simulink model "TEST_LIDAR"  (R2022b)
settings: Solver=FixedStepAuto  StartTime=0.0  StopTime=inf  FixedStep=1e-3  RelTol=1e-3  EnableMultiTasking=on
model workspace (MAT data in the model file):
  SL_ROS_VariableLengthArrays_MaxSizes.CommonInfo.ArrayTruncateAction = 'EmitWarning'
  SL_ROS_VariableLengthArrays_MaxSizes.MsgTypeMap = containers.Map
  SL_ROS_VariableLengthArrays_MaxSizes.MsgTypeMap.serialization.keys = {'sensor_msgs/LaserScan', 'time_custom_msgs/Tiempos'}
  SL_ROS_VariableLengthArrays_MaxSizes.MsgTypeMap.serialization.values{1}(1).PropertyName = 'intensities'
  SL_ROS_VariableLengthArrays_MaxSizes.MsgTypeMap.serialization.values{1}(1).DataType = 'single'
  SL_ROS_VariableLengthArrays_MaxSizes.MsgTypeMap.serialization.values{1}(1).MaxLength = 128
  SL_ROS_VariableLengthArrays_MaxSizes.MsgTypeMap.serialization.values{1}(2).PropertyName = 'ranges'
  SL_ROS_VariableLengthArrays_MaxSizes.MsgTypeMap.serialization.values{1}(2).DataType = 'single'
  SL_ROS_VariableLengthArrays_MaxSizes.MsgTypeMap.serialization.values{1}(2).MaxLength = 1
  SL_ROS_VariableLengthArrays_MaxSizes.MsgTypeMap.serialization.values{2}.PropertyName = 'data'
  SL_ROS_VariableLengthArrays_MaxSizes.MsgTypeMap.serialization.values{2}.DataType = 'uint8'
  SL_ROS_VariableLengthArrays_MaxSizes.MsgTypeMap.serialization.values{2}.MaxLength = 1400
  SL_ROS_VariableLengthArrays_MaxSizes.MsgTypeMap.serialization.uniformity = 0
  SL_ROS_VariableLengthArrays_MaxSizes.MsgTypeMap.serialization.keyType = 'char'
  SL_ROS_VariableLengthArrays_MaxSizes.MsgTypeMap.serialization.valueType = 'any'
values from neighbouring files (symbols this model uses):
  data = theClient.GetLastFrameOfData()    [FuncMotive.m]
undefined symbols (not defined in the file or in its folder): angular, carstamp, CIRCUIT, CLTF_DAMP, CLTF_FREQ, CLTF_GAIN, CONTROL, CONTROL_INI, DiscIntNeverNeededParam, INPUT, linear, MCP3201, MD25, MODEL, MODEL_INI, mpcstate, MPU60X0, MPU9250, MSG, NAV_MPC_CONTROL, OUTPUT, RCRX, SAMPLING_TIME, SYSID_INPUT, VL6180X
libraries: raspberrypiCommlib x160, simulink x89, raspberrypiNetworklib x22, ros2lib x14, dspsigattribs x14, embedlinuxBasiclib x12, ctrlSharedLib x2, mpclib x1, vrlib x1, sldrtlib x1
(part 1 of 19)
settings Model: SimulationMode=external  PauseTimes=430  ExtModeTrigDuration=2  Creator=The MathWorks, Inc.  LastModifiedBy=diego
settings SolverCC: AlgebraicLoopSolver=TrustRegion  PositivePriorityOrder=on  AutoInsertRateTranBlk=on
settings DataIOCC: LimitDataPoints=on  SaveOutput=off  SignalLogging=off  DSMLogging=off  SaveTime=off  ReturnWorkspaceOutputs=off
settings OptimizationCC: BlockReduction=off  EnhancedBackFolding=on  PassReuseOutputArgsAs=Individual arguments  ZeroExternalMemoryAtStartup=off  ZeroInternalMemoryAtStartup=off  MaxStackSize=64  OptimizeBlockOrder=speed  DifferentSizesBufferReuse=on  OptimizationCustomize=off  EfficientTunableParamExpr=on
settings DebuggingCC: MultiTaskDSMMsg=none  ParameterPrecisionLossMsg=none  ParameterTunabilityLossMsg=error  UnconnectedInputMsg=warning  UnconnectedOutputMsg=warning  UnconnectedLineMsg=warning  AllowSymbolicDim=off  PregeneratedLibrarySubsystemCodeDiagnostic=none  SFUnexpectedBacktrackingDiag=warning  SFNoUnconditionalDefaultTransitionDiag=warning  SFExecutionAtInitializationDiag=none  SFMachineParentedDataDiag=warning  ArithmeticOperatorsInVariantConditions=warning
settings HardwareCC: ProdBitPerPointer=32  ProdBitPerSizeT=32  ProdBitPerPtrDiffT=32  ProdLargestAtomicInteger=Long  ProdLargestAtomicFloat=Double  ProdWordSize=32  ProdLongLongMode=on  ProdHWDeviceType=ARM Compatible->ARM Cortex
settings ModelReferenceCC: EnableRefExpFcnMdlSchedulingChecks=on  PropagateSignalLabelsOutOfModel=off
settings SFSimCC: SimUseLocalCustomCode=off  CustomCodeUndefinedFunction=UseInterfaceOnly
settings RTWCC: Description=Embedded Coder  SystemTargetFile=ert.tlc  HardwareBoard=Raspberry Pi  TemplateMakefile=ert_default_tmf  RTWUseLocalCustomCode=off  Toolchain=GNU GCC Embedded Linux  BuildConfiguration=Faster Runs  DLArmComputeVersion=19.05
settings CodeAppCC: ForceParamTrailComments=on  IgnoreCustomStorageClasses=off  MaxIdLength=95  OperatorAnnotations=on  SimulinkDataObjDesc=on  SFDataObjDesc=on  MangleLength=10  InsertBlockDesc=on
settings ERTTargetCC: SupportVariableSizeSignals=on  ExtMode=on  ExtModeTransport=2  ExtModeStaticAlloc=on  ExtModeMexFile=ext_xcp  ExtModeMexArgs='192.168.0.103' 0 17725  ExtModeIntrfLevel=Level2 - Open
settings ConfigComp: CovMetricSettings=dw  CovSaveCumulativeToWorkspaceVar=on  CovSaveSingleToWorkspaceVar=on  CovExternalEMLEnable=off

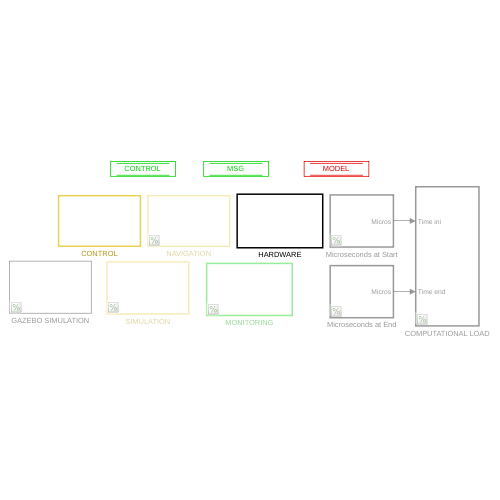
[thumbnail: Simulink's stored preview of the top-level diagram]
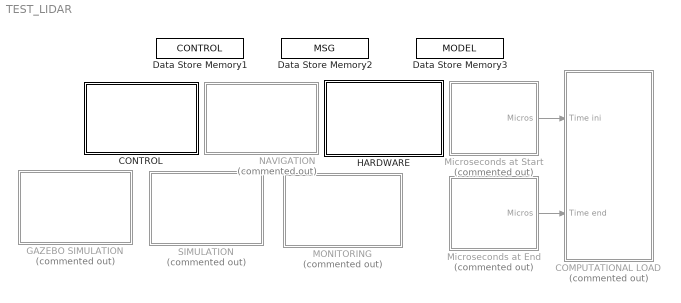
== system TEST_LIDAR ==
  COMPUTATIONAL LOAD : Subsystem  Priority=1100  Commented=on  TreatAsAtomicUnit=on  mask{Ts=SAMPLING_TIME}
      mask prompts: Ts "Sampling Time (s)"
      settings: MinAlgLoopOccurrences=on
  CONTROL : Subsystem  Priority=30  TreatAsAtomicUnit=on
      settings: MinAlgLoopOccurrences=on  RTWSystemCode=Nonreusable function  RTWFcnNameOpts=Use subsystem name  RTWFileNameOpts=Use subsystem name  FunctionWithSeparateData=on
  Data Store Memory1 : DataStoreMemory  Priority=2  DataStoreName=CONTROL  ReadBeforeWriteMsg=warning  WriteAfterWriteMsg=warning  WriteAfterReadMsg=warning  InitialValue=CONTROL_INI  ShowAdditionalParam=off  OutDataTypeStr=Bus: CONTROL_Bus
  Data Store Memory2 : DataStoreMemory  Priority=2  DataStoreName=MSG  ReadBeforeWriteMsg=warning  WriteAfterWriteMsg=warning  WriteAfterReadMsg=warning  InitialValue=MSG_INI  ShowAdditionalParam=off  OutDataTypeStr=Bus: MSG_Bus
  Data Store Memory3 : DataStoreMemory  Priority=2  DataStoreName=MODEL  ReadBeforeWriteMsg=warning  WriteAfterWriteMsg=warning  WriteAfterReadMsg=warning  InitialValue=MODEL_INI  ShowAdditionalParam=off  OutDataTypeStr=Bus: MODEL_Bus
  GAZEBO SIMULATION : Subsystem  Commented=on
  HARDWARE : Subsystem  Priority=10  TreatAsAtomicUnit=on
      settings: MinAlgLoopOccurrences=on
  MONITORING : Subsystem  Priority=100  Commented=on  TreatAsAtomicUnit=on
      settings: MinAlgLoopOccurrences=on
  Microseconds at End : Subsystem  Priority=1000  Commented=on  TreatAsAtomicUnit=on
      settings: MinAlgLoopOccurrences=on
  Microseconds at Start : Subsystem  Priority=0  Commented=on  TreatAsAtomicUnit=on
      settings: MinAlgLoopOccurrences=on
  NAVIGATION : Subsystem  Priority=30  Commented=on  TreatAsAtomicUnit=on
      settings: MinAlgLoopOccurrences=on  RTWSystemCode=Nonreusable function  RTWFcnNameOpts=Use subsystem name  RTWFileNameOpts=Use subsystem name  FunctionWithSeparateData=on
  SIMULATION : Subsystem  Priority=10  Commented=on  TreatAsAtomicUnit=on
      settings: MinAlgLoopOccurrences=on
  wires:
  Microseconds at End/1(Micros) -> COMPUTATIONAL LOAD/2(Time end)
  Microseconds at Start/1(Micros) -> COMPUTATIONAL LOAD/1(Time ini)

== system TEST_LIDAR/COMPUTATIONAL LOAD ==
  Time ini : Inport
  Time end : Inport  Port=2
  Accumulator 1 : Subsystem
  Accumulator 2 : Subsystem
  Accumulator 3 : Subsystem
  Accumulator 4 : Subsystem
  CPU Utilization (%) : Display
  CPU time (s) : Display
  Compare To Constant : simulink/Logic and Bit Operations/Compare To Constant  relop=>=  const=100  OutDataTypeStr=uint8
  Compare To Constant1 : simulink/Logic and Bit Operations/Compare To Constant  relop=>=  const=0  OutDataTypeStr=uint8
  Compare To Constant2 : simulink/Logic and Bit Operations/Compare To Constant  relop=<  const=0  OutDataTypeStr=uint8
  Cycles : Display
  Cycles Over 100% : Display
  Data Store Write : DataStoreWrite  DataStoreName=CONTROL  DataStoreElements=CONTROL.STATE.CPU_LOAD  IndexOptions=Index vector (dialog)  Indices=1  OutputSizes=1
  Data Type Conversion : DataTypeConversion  OutDataTypeStr=single  SaturateOnIntegerOverflow=off  RndMeth=Floor
  Data Type Conversion1 : DataTypeConversion  OutDataTypeStr=single  SaturateOnIntegerOverflow=off  RndMeth=Floor
  Data Type Conversion3 : DataTypeConversion  OutDataTypeStr=uint8  SaturateOnIntegerOverflow=off  RndMeth=Floor
  Gain : Gain  Gain=1e-4/Ts
  Gain1 : Gain  Gain=1e6
  Gain2 : Gain  Gain=1e3
  Mux2 : Mux  Inputs=2
  "Probably, priority error or time overflow" : Display
  Sum : Sum  Inputs=-|+  OutDataTypeStr=double
  usecs per Ts : Constant  Value=Ts*1e6  SampleTime=Ts
  wires:
  usecs per Ts/1 -> Accumulator 1/1(In)
  Sum/1 -> Gain/1
  Time ini/1 -> Gain2/1, Sum/1
  Accumulator 1/1(Sum) -> Gain1/1
  Accumulator 3/1(Sum) -> Cycles/1
  Compare To Constant1/1 -> Accumulator 3/1(In)
  Accumulator 2/1(Sum) -> Cycles Over 100%/1
  Compare To Constant/1 -> Accumulator 2/1(In)
  Time end/1 -> Sum/2
  Gain/1 -> CPU Utilization (%)/1, Data Type Conversion3/1, Compare To Constant/1, Compare To Constant2/1, Compare To Constant1/1
  Compare To Constant2/1 -> Accumulator 4/1(In)
  Accumulator 4/1(Sum) -> "Probably, priority error or time overflow"/1
  Gain1/1 -> Data Type Conversion/1
  Gain2/1 -> Data Type Conversion1/1
  Data Type Conversion/1 -> Mux2/1
  Data Type Conversion1/1 -> Mux2/2
  Mux2/1 -> CPU time (s)/1
  Data Type Conversion3/1 -> Data Store Write/1

== system TEST_LIDAR/CONTROL ==
  ACCELERATION RATE : Subsystem  Priority=50  Commented=on  TreatAsAtomicUnit=on
      settings: MinAlgLoopOccurrences=on
  ADAPTIVE CONTROL STR : Subsystem  Priority=200  Commented=on
      settings: MinAlgLoopOccurrences=on
  "CONTROL UPDATE " : MATLAB Function  Priority=30  Commented=on  TreatAsAtomicUnit=on
      settings: MinAlgLoopOccurrences=on
  Compare To Constant4 : simulink/Logic and Bit Operations/Compare To Constant  Commented=on  relop=>  const=0  OutDataTypeStr=boolean
  Compare To Constant9 : simulink/Logic and Bit Operations/Compare To Constant  Commented=on  relop===  const=5  OutDataTypeStr=boolean
  Data Store Read1 : DataStoreRead  Commented=on  DataStoreName=CONTROL  SampleTime=SAMPLING_TIME  IndexOptions=Index vector (dialog)  Indices=1  OutputSizes=1
  Data Store Read10 : DataStoreRead  Commented=on  DataStoreName=CONTROL  SampleTime=SAMPLING_TIME  DataStoreElements=CONTROL.OUTPUT.MOTOR_VOLT(:,:)  IndexOptions=Index vector (dialog)  Indices=1  OutputSizes=1
  Data Store Read11 : DataStoreRead  Commented=on  DataStoreName=CONTROL  SampleTime=SAMPLING_TIME  DataStoreElements=CONTROL.INPUT.BATTERY_VOLT  IndexOptions=Index vector (dialog)  Indices=1  OutputSizes=1
  Data Store Read2 : DataStoreRead  Commented=on  DataStoreName=CONTROL  SampleTime=SAMPLING_TIME  IndexOptions=Index vector (dialog)  Indices=1  OutputSizes=1
  Data Store Read5 : DataStoreRead  DataStoreName=MSG  SampleTime=SAMPLING_TIME  IndexOptions=Index vector (dialog)  Indices=1  OutputSizes=1
  Data Store Read6 : DataStoreRead  Commented=on  DataStoreName=CONTROL  SampleTime=SAMPLING_TIME  DataStoreElements=CONTROL.STATE.CURRENT_STATUS_SYS  IndexOptions=Index vector (dialog)  Indices=1  OutputSizes=1
  Data Store Read7 : DataStoreRead  DataStoreName=CONTROL  SampleTime=SAMPLING_TIME  IndexOptions=Index vector (dialog)  Indices=1  OutputSizes=1
  Data Store Read8 : DataStoreRead  Commented=on  DataStoreName=CONTROL  SampleTime=SAMPLING_TIME  DataStoreElements=CONTROL.STATE.STR_MODE  IndexOptions=Index vector (dialog)  Indices=1  OutputSizes=1
  Data Store Read9 : DataStoreRead  Commented=on  DataStoreName=CONTROL  SampleTime=SAMPLING_TIME  DataStoreElements=CONTROL.STATE.CONTROL_STATUS  IndexOptions=Index vector (dialog)  Indices=1  OutputSizes=1
  Data Store Write : DataStoreWrite  Commented=on  DataStoreName=CONTROL  DataStoreElements=CONTROL.OUTPUT.REAL_MOTOR_VOLT(:,:)  IndexOptions=Index vector (dialog)  Indices=1  OutputSizes=1
  Data Store Write1 : DataStoreWrite  Commented=on  DataStoreName=CONTROL  IndexOptions=Index vector (dialog)  Indices=1  OutputSizes=1
  Data Store Write2 : DataStoreWrite  Commented=on  DataStoreName=CONTROL  IndexOptions=Index vector (dialog)  Indices=1  OutputSizes=1
  Data Store Write3 : DataStoreWrite  DataStoreName=CONTROL  IndexOptions=Index vector (dialog)  Indices=1  OutputSizes=1
  Data Store Write5 : DataStoreWrite  DataStoreName=MSG  IndexOptions=Index vector (dialog)  Indices=1  OutputSizes=1
  Data Store Write6 : DataStoreWrite  Commented=on  DataStoreName=CONTROL  DataStoreElements=CONTROL.OUTPUT.REAL_MOTOR_VOLT_CD(:,:)  IndexOptions=Index vector (dialog)  Indices=1  OutputSizes=1
  LOCAL TARGETS : Subsystem  Priority=5  Commented=on  TreatAsAtomicUnit=on
      settings: MinAlgLoopOccurrences=on
  Logical Operator1 : Logic  Commented=on  AllPortsSameDT=off  OutDataTypeStr=boolean
  MOTOR DELAY : Subsystem  Priority=40  Commented=on  TreatAsAtomicUnit=on
      settings: MinAlgLoopOccurrences=on
  STATE ESTIMATOR : MATLAB Function  Priority=20  Commented=on  TreatAsAtomicUnit=on
      settings: MinAlgLoopOccurrences=on
  STATE MACHINE UPDATE : MATLAB Function  Priority=1000  TreatAsAtomicUnit=on
      settings: MinAlgLoopOccurrences=on
  SYSTEM IDENTIFICATION : Subsystem  Priority=150  Commented=on  TreatAsAtomicUnit=on
      mask init:
      | %%%%%%%%%%%%%%%%%%%%%%%%%%%%%%%%%%%%%%%%%%%%%%%%%%%%%%
      | %%  STATE VARIABLE FILTER FOR SYSTEM IDENTIFICATION  %
      | %%%%%%%%%%%%%%%%%%%%%%%%%%%%%%%%%%%%%%%%%%%%%%%%%%%%%%
      | % Natural frequency (rad/s)
      | SVF_FREQ = 10;
      | % Factor defining band pass width
      | SVF_FACTOR = 5;
      | % FILTER ORDER/2
      | SVF_ORD = 2;
      | % Km/(Tm*Tf*s^2 + (Tm+Tf)*s + 1) = Km/Tm/Tf/(s^2 + (Tm+Tf)/Tm/Tf*s + 1/Tm/Tf)
      | % b0/(s^2 + a1*s + a0)
      | % D2y + a1*D1y + a0*y = b0*u
      | % D1y + a1*y + a0*I1y = b0*I1u
      | % D1yf = - a1*yf - a0*I1y + b0I1uf
      | %  -a1=-(Tm+Tf)/Tm/Tf / -a0=-1/Tm/Tf / b0=Km/Tm/Tf 
      | % Butterworh filter desig
      | [SVF_NUM,SVF_DEN]=butter(SVF_ORD,[SVF_FREQ/SVF_FACTOR SVF_FACTOR*SVF_FREQ],'s');
      | % Controlability canonical-form 
      | SVF_A = single([zeros(2*SVF_ORD-1,1) eye(2*SVF_ORD-1) ; -SVF_DEN(end:-1:2)]);
      | SVF_B = single([zeros(2*SVF_ORD-1,1) ; SVF_NUM(end-SVF_ORD)]);
      | % Sampling time
      | ts = 10e-3;
      | % Triangular hold
      | % x[k] = Ad*x[k-1] + B1d*u[k-1] + B2d*u[k]
      | % Ad = expm(A*ts)
      | % B1d = A\(Ad+inv(A)/ts-inv(A)*Ad/ts)*B;
      | % B2d = A\(inv(A)*Ad/ts-eye(2)-inv(A)/ts)*B;
      | SVF_Ad = expm(SVF_A*ts);
      | SVF_B1d = SVF_A\(SVF_Ad+inv(SVF_A)/ts-SVF_A\SVF_Ad/ts)*SVF_B;
      | SVF_B2d = SVF_A\(SVF_A\SVF_Ad/ts-eye(2*SVF_ORD)-inv(SVF_A)/ts)*SVF_B;
      settings: MinAlgLoopOccurrences=on
  wires:
  STATE MACHINE UPDATE/1(CONTROL) -> Data Store Write3/1
  STATE ESTIMATOR/1(CONTROL) -> Data Store Write2/1
  "CONTROL UPDATE "/1(CONTROL) -> Data Store Write1/1
  Data Store Read2/1 -> STATE ESTIMATOR/1(CONTROL_IN)
  STATE MACHINE UPDATE/2(MSG) -> Data Store Write5/1
  Data Store Read5/1 -> STATE MACHINE UPDATE/2(MSG_IN)
  Data Store Read8/1 -> Logical Operator1/2
  Logical Operator1/1 -> ADAPTIVE CONTROL STR/Enable
  Data Store Read6/1 -> Compare To Constant9/1
  Compare To Constant9/1 -> Logical Operator1/1
  SYSTEM IDENTIFICATION/1(VEL_PARAM) -> ADAPTIVE CONTROL STR/1(VEL_PARAM)
  "CONTROL UPDATE "/3(MOTOR_VOLT_CD) -> MOTOR DELAY/2(MOTOR_VOLT_CD)
  Data Store Read1/1 -> "CONTROL UPDATE "/1(CONTROL_IN)
  Data Store Read7/1 -> STATE MACHINE UPDATE/1(CONTROL_IN)
  "CONTROL UPDATE "/2(MOTOR_VOLT) -> MOTOR DELAY/1(MOTOR_VOLT)
  Data Store Read9/1 -> Compare To Constant4/1
  Compare To Constant4/1 -> LOCAL TARGETS/Enable
  Data Store Read11/1 -> ACCELERATION RATE/2(MOTOR VOLT MAX)
  Data Store Read10/1 -> ACCELERATION RATE/1(CONTROL MOTOR VOLT)
  ACCELERATION RATE/1(REAL MOTOR VOLT) -> Data Store Write/1
  ACCELERATION RATE/2(REAL MOTOR VOLT_CD) -> Data Store Write6/1

== system TEST_LIDAR/GAZEBO SIMULATION ==
  BUTTON_A : Constant  Commented=on  Value=0  OutDataTypeStr=uint8  SampleTime=SAMPLING_TIME
  BUTTON_B : Constant  Commented=on  Value=0  OutDataTypeStr=uint8  SampleTime=SAMPLING_TIME
  BUTTON_C : Constant  Commented=on  Value=0  OutDataTypeStr=uint8  SampleTime=SAMPLING_TIME
  Bus Assignment : BusAssignment  Priority=40  Commented=on  AssignedSignals=STATE.BUTTONS
  COMMUNICATIONS : Subsystem
      settings: MinAlgLoopOccurrences=on
  Cast : DataTypeConversion  Commented=on  OutDataTypeStr=uint8  SaturateOnIntegerOverflow=off  RndMeth=Floor
  Data Store Read1 : DataStoreRead  Commented=on  DataStoreName=CONTROL  SampleTime=SAMPLING_TIME  DataStoreElements=CONTROL.STATE.BUTTONS(:,:)  IndexOptions=Index vector (dialog)  Indices=1  OutputSizes=1
  Data Store Read5 : DataStoreRead  Commented=on  DataStoreName=CONTROL  SampleTime=SAMPLING_TIME  DataStoreElements=CONTROL.STATE.PC_BUTTONS(:,:)  IndexOptions=Index vector (dialog)  Indices=1  OutputSizes=1
  Data Store Read9 : DataStoreRead  Commented=on  DataStoreName=CONTROL  SampleTime=SAMPLING_TIME  IndexOptions=Index vector (dialog)  Indices=1  OutputSizes=1
  Data Store Write4 : DataStoreWrite  Commented=on  DataStoreName=CONTROL  IndexOptions=Index vector (dialog)  Indices=1  OutputSizes=1
  Logical Operator : Logic  Commented=on  Operator=OR  Inputs=3  AllPortsSameDT=off  OutDataTypeStr=boolean
  Mux : Mux  Commented=on  Inputs=3
  Push Button3 : PushButtonBlock  Commented=on  ButtonText=BUTTON A  OffValue=0.000000
  Push Button4 : PushButtonBlock  Commented=on  ButtonText=BUTTON B  OffValue=0.000000
  Push Button5 : PushButtonBlock  Commented=on  ButtonText=BUTTON C  OffValue=0.000000
  SEND MOTOR VOLTAGE : Subsystem
  SENSORS : Subsystem
  wires:
  Data Store Read9/1 -> Bus Assignment/1
  BUTTON_C/1 -> Mux/3
  BUTTON_B/1 -> Mux/2
  Mux/1 -> Logical Operator/1
  Data Store Read1/1 -> Logical Operator/3
  Data Store Read5/1 -> Logical Operator/2
  Cast/1 -> Bus Assignment/2
  Logical Operator/1 -> Cast/1
  BUTTON_A/1 -> Mux/1
  Bus Assignment/1 -> Data Store Write4/1

== system TEST_LIDAR/HARDWARE ==
  ACTUATORS : Subsystem  Priority=10  SystemSampleTime=SAMPLING_TIME
      settings: MinAlgLoopOccurrences=on  RTWSystemCode=Nonreusable function  RTWFcnNameOpts=Use subsystem name  RTWFileNameOpts=Use subsystem name  FunctionWithSeparateData=on
  COMMUNICATIONS : Subsystem
      settings: MinAlgLoopOccurrences=on
  SENSORS : Subsystem  Priority=0
      settings: MinAlgLoopOccurrences=on  RTWSystemCode=Nonreusable function  RTWFcnNameOpts=Use subsystem name  RTWFileNameOpts=Use subsystem name  FunctionWithSeparateData=on

== system TEST_LIDAR/MONITORING ==
  BLACKBOX : Subsystem  Priority=20  TreatAsAtomicUnit=on
      settings: MinAlgLoopOccurrences=on
  COMMUNICATIONS : Subsystem  Priority=0  TreatAsAtomicUnit=on
      settings: MinAlgLoopOccurrences=on  RTWSystemCode=Nonreusable function  RTWFcnNameOpts=Use subsystem name  RTWFileNameOpts=Use subsystem name  FunctionWithSeparateData=on
  EXTERNAL MODE: SCOPES : Subsystem  Priority=10  Commented=on  TreatAsAtomicUnit=on
      settings: MinAlgLoopOccurrences=on
  FV COMPETITION: SCOPES : Subsystem  Commented=on  TreatAsAtomicUnit=on
      settings: MinAlgLoopOccurrences=on
  HARDWARE: SCOPES : Subsystem  Priority=1000  Commented=on
  NAV COMPETITION: SCOPES : Subsystem  Priority=20  Commented=on  TreatAsAtomicUnit=on
      settings: MinAlgLoopOccurrences=on
  ROS_COM : Subsystem  Priority=0  Commented=on  TreatAsAtomicUnit=on
      settings: MinAlgLoopOccurrences=on  RTWSystemCode=Nonreusable function  RTWFcnNameOpts=Use subsystem name  RTWFileNameOpts=Use subsystem name  FunctionWithSeparateData=on
  SIMULATION: SCOPES : Subsystem  Priority=40  Commented=on
  TEST: SCOPES : Subsystem  Priority=40  Commented=on  TreatAsAtomicUnit=on
      settings: MinAlgLoopOccurrences=on

== system TEST_LIDAR/Microseconds at End ==
  Microseconds_or : S-Function  InitFcn=try, set_param(gcb,'FunctionName','sfcn_micros'), end  FunctionName=sfcn_micros  SFunctionModules=sfcn_micros_wrapper.c  SFunctionDeploymentMode=off  EnableBusSupport=off  mask(S-Function Builder){}
      mask init:
      | val = [[.9  0.75 0.75 1 1 .9 .9 1]',[1 1 0.75 0.75 .9 .9 1 .9]'];try , sys = get_param(gcb,'SfunBuilderFcnName');if isempty(sys), sys = get_param(gcb,'FunctionName'); end,catch, sys = get_param(gcb,'FunctionName'); end
      settings: CopyFcn=set_param(gcbh,'LinkStatus','none')  PreSaveFcn=try, set_param(gcb,'FunctionName','sfcn_micros'), end  OpenFcn=sfunctionwizard(gcbh)
      mask Display: plot(val(:,1),val(:,2)),disp(sys), port_label('output',1,'microseconds')
  Micros : Outport  VectorParamsAs1DForOutWhenUnconnected=off
  wires:
  Microseconds_or/1 -> Micros/1

== system TEST_LIDAR/Microseconds at Start ==
  Microseconds_or : S-Function  InitFcn=try, set_param(gcb,'FunctionName','sfcn_micros'), end  FunctionName=sfcn_micros  SFunctionModules=sfcn_micros_wrapper  SFunctionDeploymentMode=off  EnableBusSupport=off  mask(S-Function Builder){}
      mask init: same as TEST_LIDAR/Microseconds at End/Microseconds_or
      settings: CopyFcn=set_param(gcbh,'LinkStatus','none')  PreSaveFcn=try, set_param(gcb,'FunctionName','sfcn_micros'), end  OpenFcn=sfunctionwizard(gcbh)
      mask Display: plot(val(:,1),val(:,2)),disp(sys), port_label('output',1,'microseconds')
  Micros : Outport  VectorParamsAs1DForOutWhenUnconnected=off
  wires:
  Microseconds_or/1 -> Micros/1

== system TEST_LIDAR/NAVIGATION ==
  Bus Assignment : BusAssignment  Commented=on  AssignedSignals=TARGET.ATT_REF
  Compare To Constant1 : simulink/Logic and Bit Operations/Compare To Constant  Commented=on  relop=>  const=1  OutDataTypeStr=boolean
  Compare To Constant11 : simulink/Logic and Bit Operations/Compare To Constant  Commented=on  relop===  const=9  OutDataTypeStr=boolean
  Compare To Constant12 : simulink/Logic and Bit Operations/Compare To Constant  Commented=on  relop===  const=6  OutDataTypeStr=boolean
  Compare To Constant3 : simulink/Logic and Bit Operations/Compare To Constant  Commented=on  relop=>  const=1  OutDataTypeStr=boolean
  Data Store Read : DataStoreRead  Commented=on  DataStoreName=CONTROL  SampleTime=SAMPLING_TIME  IndexOptions=Index vector (dialog)  Indices=1  OutputSizes=1
  Data Store Read3 : DataStoreRead  Commented=on  DataStoreName=CONTROL  SampleTime=SAMPLING_TIME  DataStoreElements=CONTROL.STATE.CONTROL_MODE#CONTROL.STATE.CONTROL_STATUS  IndexOptions=Index vector (dialog)  Indices=1  OutputSizes=1
  Data Store Read4 : DataStoreRead  Commented=on  DataStoreName=CONTROL  SampleTime=SAMPLING_TIME  IndexOptions=Index vector (dialog)  Indices=1  OutputSizes=1
  Data Store Read5 : DataStoreRead  Commented=on  DataStoreName=CONTROL  SampleTime=SAMPLING_TIME  DataStoreElements=CONTROL.STATE.CURRENT_STATUS_SYS  IndexOptions=Index vector (dialog)  Indices=1  OutputSizes=1
  Data Store Write4 : DataStoreWrite  Commented=on  DataStoreName=CONTROL  IndexOptions=Index vector (dialog)  Indices=1  OutputSizes=1
  Logical Operator : Logic  Commented=on  AllPortsSameDT=off  OutDataTypeStr=boolean
  Logical Operator2 : Logic  Commented=on  Operator=OR  AllPortsSameDT=off  OutDataTypeStr=boolean
  MPC CONTROL FOR NAVIGATION VELOCITY MAGNITUDE AND ANGLE : Subsystem  Priority=30  Commented=on
  NAVIGATION TARGETS : Subsystem  Priority=10  Commented=on
      settings: MinAlgLoopOccurrences=on
  Rate Transition : RateTransition  Commented=on  OutPortSampleTime=CONTROL_INI.PARAM.NAV_MPC.SAMPLING_TIME
  Rate Transition1 : RateTransition  Commented=on  OutPortSampleTime=SAMPLING_TIME
  Rate Transition2 : RateTransition  Commented=on  OutPortSampleTime=CONTROL_INI.PARAM.NAV_MPC.SAMPLING_TIME
  wires:
  Data Store Read3/1 -> Compare To Constant3/1
  Data Store Read3/2 -> Compare To Constant1/1
  Compare To Constant3/1 -> Logical Operator/1
  Compare To Constant1/1 -> Logical Operator/2
  Logical Operator/1 -> Rate Transition2/1
  MPC CONTROL FOR NAVIGATION VELOCITY MAGNITUDE AND ANGLE/1(Output) -> Rate Transition1/1
  Bus Assignment/1 -> Data Store Write4/1
  Data Store Read/1 -> Bus Assignment/1
  Data Store Read4/1 -> Rate Transition/1
  Rate Transition/1 -> MPC CONTROL FOR NAVIGATION VELOCITY MAGNITUDE AND ANGLE/1(Input)
  Rate Transition1/1 -> Bus Assignment/2
  Rate Transition2/1 -> MPC CONTROL FOR NAVIGATION VELOCITY MAGNITUDE AND ANGLE/Enable
  Logical Operator2/1 -> NAVIGATION TARGETS/Enable
  Compare To Constant11/1 -> Logical Operator2/2
  Compare To Constant12/1 -> Logical Operator2/1
  Data Store Read5/1 -> Compare To Constant11/1, Compare To Constant12/1

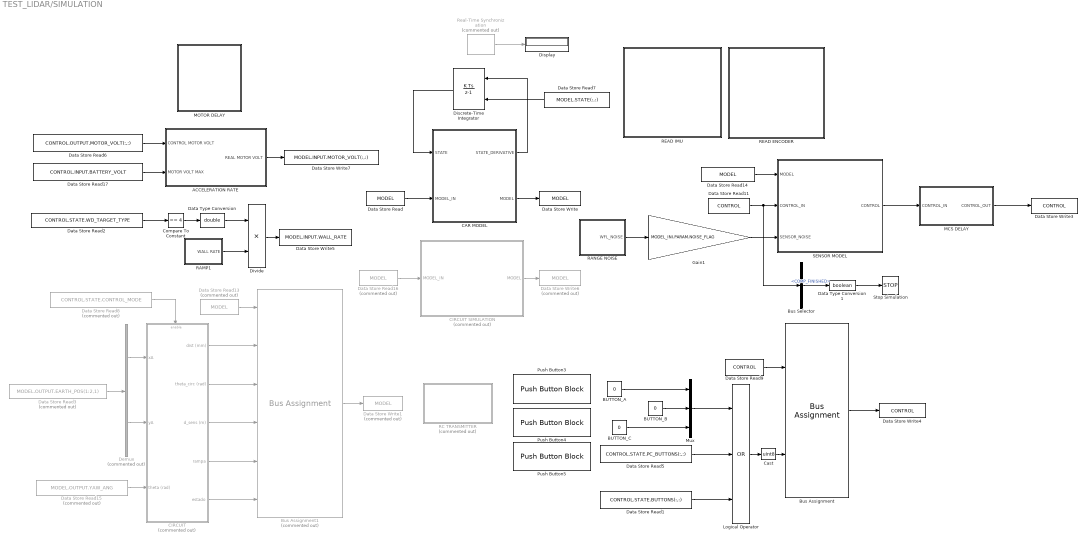
== system TEST_LIDAR/SIMULATION ==
  ACCELERATION RATE : Subsystem  Priority=0
  BUTTON_A : Constant  Value=0  OutDataTypeStr=uint8  SampleTime=SAMPLING_TIME
  BUTTON_B : Constant  Value=0  OutDataTypeStr=uint8  SampleTime=SAMPLING_TIME
  BUTTON_C : Constant  Value=0  OutDataTypeStr=uint8  SampleTime=SAMPLING_TIME
  Bus Assignment : BusAssignment  Priority=40  AssignedSignals=STATE.BUTTONS
  Bus Assignment1 : BusAssignment  Commented=on  AssignedSignals=OUTPUT.RANGE_WALL_DIST,OUTPUT.RANGE_YAW_ANG,OUTPUT.RANGE_SENS,CIRCUIT.RAMP,CIRCUIT.STATUS
  Bus Selector : BusSelector  OutputSignals=STATE.COMP_FINISHED
  "CAR MODEL " : MATLAB Function  Priority=30  TreatAsAtomicUnit=on
      settings: MinAlgLoopOccurrences=on
  CIRCUIT : Subsystem  Commented=on  mask{N=MODEL_INI.CIRCUIT.PERIMETER_POINTS, L=MODEL_INI.CIRCUIT.STRAIGHT_SIDE_LENGTH, Lr=MODEL_INI.CIRCUIT.RAMP_LENGTH, R=MODEL_INI.CIRCUIT.CURVE_RADIUS, d_sens=MODEL_INI.PARAM.RANGE_SENS_DIST, ts=MODEL_INI.PARAM.SIM_SAMPLING_TIME}
      mask prompts: N "Numero de puntos para generar el perimetro"; L "Longitud del tramo recto (m)"; Lr "Longitud rampa (m)"; R "Radio de la curva (m)"; d_sens "Distancia entre sensores (m)"; ts "Período de muestreo (s)"
      mask init:
      | %% SISTEMA DE REFERENCIA INERCIAL
      | % El origen de coordenadas esta justo en la mitad del circuito
      | % Eje X paralelo al tramo recto en el sentido de la marcha y eje Y perpedicular
      | % Ecuacion de los tramos rectos
      | % y = R para -L/2 < x < L/2
      | % y = -R para -L/2 < x < L/2
      | % (x-L/2)^2 + y^2 = R^2  para x > L/2
      | % (x+L/2)^2 + y^2 = R^2  para x < -L/2
      | % Calculo de la secuencia de puntos
      | % aux=pi/2/floor(N/4);
      | % X_circ=[-R*cos(linspace(aux,pi/2-aux,floor(N/4)))-L/2 ...
      | %         linspace(-L/2,L/2,floor(N/2)) ...
      | %         R*sin(linspace(aux,pi/2-aux,floor(N/4)))+L/2];
      | % Y_circ=-R*(X_circ>=-L/2 & X_circ<=L/2)-...
      | %         sqrt(R^2-(X_circ-L/2).^2).*(X_circ>L/2)+...
      | %         -sqrt(R^2-(X_circ+L/2).^2).*(X_circ<-L/2);
      | % Y_circ=[Y_circ(:) ; -flipud(Y_circ(:))];
      | % X_circ=[X_circ(:) ; flipud(X_circ(:))];
      | 
      | % parametros
      | param=[L Lr R d_sens];
  CIRCUIT SIMULATION : MATLAB Function  Commented=on  TreatAsAtomicUnit=on
  Cast : DataTypeConversion  OutDataTypeStr=uint8  SaturateOnIntegerOverflow=off  RndMeth=Floor
  Compare To Constant : simulink/Logic and Bit Operations/Compare To Constant  relop===  const=4  OutDataTypeStr=uint8
  Data Store Read : DataStoreRead  DataStoreName=MODEL  SampleTime=MODEL_INI.PARAM.SIM_SAMPLING_TIME  IndexOptions=Index vector (dialog)  Indices=1  OutputSizes=1
  Data Store Read1 : DataStoreRead  DataStoreName=CONTROL  SampleTime=SAMPLING_TIME  DataStoreElements=CONTROL.STATE.BUTTONS(:,:)  IndexOptions=Index vector (dialog)  Indices=1  OutputSizes=1
  Data Store Read11 : DataStoreRead  DataStoreName=CONTROL  SampleTime=SAMPLING_TIME  IndexOptions=Index vector (dialog)  Indices=1  OutputSizes=1
  Data Store Read13 : DataStoreRead  Commented=on  DataStoreName=MODEL  SampleTime=0  IndexOptions=Index vector (dialog)  Indices=1  OutputSizes=1
  Data Store Read14 : DataStoreRead  Priority=30  DataStoreName=MODEL  SampleTime=SAMPLING_TIME  IndexOptions=Index vector (dialog)  Indices=1  OutputSizes=1
  Data Store Read15 : DataStoreRead  Commented=on  DataStoreName=MODEL  SampleTime=MODEL_INI.PARAM.SAMPLING_TIME  DataStoreElements=MODEL.OUTPUT.YAW_ANG  IndexOptions=Index vector (dialog)  Indices=1  OutputSizes=1
  Data Store Read16 : DataStoreRead  Commented=on  DataStoreName=MODEL  SampleTime=MODEL_INI.PARAM.SIM_SAMPLING_TIME  IndexOptions=Index vector (dialog)  Indices=1  OutputSizes=1
  Data Store Read17 : DataStoreRead  DataStoreName=CONTROL  SampleTime=SAMPLING_TIME  DataStoreElements=CONTROL.INPUT.BATTERY_VOLT  IndexOptions=Index vector (dialog)  Indices=1  OutputSizes=1
  Data Store Read2 : DataStoreRead  DataStoreName=CONTROL  SampleTime=MODEL_INI.PARAM.SIM_SAMPLING_TIME  DataStoreElements=CONTROL.STATE.WD_TARGET_TYPE  IndexOptions=Index vector (dialog)  Indices=1  OutputSizes=1
  Data Store Read3 : DataStoreRead  Commented=on  DataStoreName=MODEL  SampleTime=MODEL_INI.PARAM.SAMPLING_TIME  DataStoreElements=MODEL.OUTPUT.EARTH_POS(1:2,1)  IndexOptions=Index vector (dialog)  Indices=1  OutputSizes=1
  Data Store Read5 : DataStoreRead  DataStoreName=CONTROL  SampleTime=SAMPLING_TIME  DataStoreElements=CONTROL.STATE.PC_BUTTONS(:,:)  IndexOptions=Index vector (dialog)  Indices=1  OutputSizes=1
  Data Store Read6 : DataStoreRead  DataStoreName=CONTROL  SampleTime=SAMPLING_TIME  DataStoreElements=CONTROL.OUTPUT.MOTOR_VOLT(:,:)  IndexOptions=Index vector (dialog)  Indices=1  OutputSizes=1
  Data Store Read7 : DataStoreRead  DataStoreName=MODEL  SampleTime=MODEL_INI.PARAM.SIM_SAMPLING_TIME  DataStoreElements=MODEL.STATE(:,:)  IndexOptions=Index vector (dialog)  Indices=1  OutputSizes=1
  Data Store Read8 : DataStoreRead  Commented=on  DataStoreName=CONTROL  SampleTime=MODEL_INI.PARAM.SIM_SAMPLING_TIME  DataStoreElements=CONTROL.STATE.CONTROL_MODE  IndexOptions=Index vector (dialog)  Indices=1  OutputSizes=1
  Data Store Read9 : DataStoreRead  DataStoreName=CONTROL  SampleTime=SAMPLING_TIME  IndexOptions=Index vector (dialog)  Indices=1  OutputSizes=1
  Data Store Write : DataStoreWrite  DataStoreName=MODEL  IndexOptions=Index vector (dialog)  Indices=1  OutputSizes=1
  Data Store Write1 : DataStoreWrite  Commented=on  DataStoreName=MODEL  IndexOptions=Index vector (dialog)  Indices=1  OutputSizes=1
  Data Store Write3 : DataStoreWrite  DataStoreName=CONTROL  IndexOptions=Index vector (dialog)  Indices=1  OutputSizes=1
  Data Store Write4 : DataStoreWrite  DataStoreName=CONTROL  IndexOptions=Index vector (dialog)  Indices=1  OutputSizes=1
  Data Store Write5 : DataStoreWrite  DataStoreName=MODEL  DataStoreElements=MODEL.INPUT.WALL_RATE  IndexOptions=Index vector (dialog)  Indices=1  OutputSizes=1
  Data Store Write6 : DataStoreWrite  Commented=on  DataStoreName=MODEL  IndexOptions=Index vector (dialog)  Indices=1  OutputSizes=1
  Data Store Write7 : DataStoreWrite  DataStoreName=MODEL  DataStoreElements=MODEL.INPUT.MOTOR_VOLT(:,:)  IndexOptions=Index vector (dialog)  Indices=1  OutputSizes=1
  Data Type Conversion : DataTypeConversion  OutDataTypeStr=double  SaturateOnIntegerOverflow=off  RndMeth=Floor
  Data Type Conversion1 : DataTypeConversion  OutDataTypeStr=boolean  SaturateOnIntegerOverflow=off  RndMeth=Floor
  Demux : Demux  Commented=on  Outputs=2
  Discrete-Time Integrator : DiscreteIntegrator  InitialConditionSource=external  SampleTime=-1  ICPrevOutput=DiscIntNeverNeededParam  ICPrevScaledInput=DiscIntNeverNeededParam
  Display : Display
  Divide : Product
  Gain1 : Gain  Gain=MODEL_INI.PARAM.NOISE_FLAG
  Logical Operator : Logic  Operator=OR  Inputs=3  AllPortsSameDT=off  OutDataTypeStr=boolean
  MCS DELAY : Subsystem  Priority=1000
  MOTOR DELAY : Subsystem  Priority=10  TreatAsAtomicUnit=on
      settings: MinAlgLoopOccurrences=on
  Mux : Mux  Inputs=3
  Push Button3 : PushButtonBlock  ButtonText=BUTTON A  OffValue=0.000000
  Push Button4 : PushButtonBlock  ButtonText=BUTTON B  OffValue=0.000000
  Push Button5 : PushButtonBlock  ButtonText=BUTTON C  OffValue=0.000000
  RAMP1 : Subsystem
  RANGE NOISE : Subsystem
  "RC TRANSMITTER " : Subsystem  Commented=on  TreatAsAtomicUnit=on  VariantControl=Variants.Command==1
      settings: MinAlgLoopOccurrences=on
  READ ENCODER : Subsystem  Priority=50
  READ IMU : Subsystem  Priority=50  TreatAsAtomicUnit=on
      settings: MinAlgLoopOccurrences=on  RTWSystemCode=Nonreusable function
  Real-Time Synchronization : sldrtlib/Real-Time Synchronization  Commented=on  SampleTime=MODEL_INI.PARAM.SIM_SAMPLING_TIME  MaxMissedTicks=10000  ShowMissedTicks=on  YieldWhenWaiting=off
  SENSOR MODEL : MATLAB Function  Priority=100  TreatAsAtomicUnit=on
  Stop Simulation : Stop
  wires:
  Data Store Read7/1 -> Discrete-Time Integrator/2
  Data Store Read/1 -> "CAR MODEL "/2(MODEL_IN)
  "CAR MODEL "/1(STATE_DERIVATIVE) -> Discrete-Time Integrator/1
  BUTTON_B/1 -> Mux/2
  Data Store Read9/1 -> Bus Assignment/1
  BUTTON_C/1 -> Mux/3
  Bus Assignment/1 -> Data Store Write4/1
  Logical Operator/1 -> Cast/1
  Mux/1 -> Logical Operator/1
  Data Store Read5/1 -> Logical Operator/2
  Cast/1 -> Bus Assignment/2
  Discrete-Time Integrator/1 -> "CAR MODEL "/1(STATE)
  BUTTON_A/1 -> Mux/1
  Real-Time Synchronization/1 -> Display/1
  Gain1/1 -> SENSOR MODEL/3(SENSOR_NOISE)
  Data Store Read14/1 -> SENSOR MODEL/1(MODEL)
  RANGE NOISE/1(WFL_NOISE) -> Gain1/1
  Data Store Read1/1 -> Logical Operator/3
  SENSOR MODEL/1(CONTROL) -> MCS DELAY/1(CONTROL_IN)
  "CAR MODEL "/2(MODEL) -> Data Store Write/1
  RAMP1/1(WALL RATE) -> Divide/2
  Divide/1 -> Data Store Write5/1
  Data Store Read2/1 -> Compare To Constant/1
  Data Type Conversion/1 -> Divide/1
  Compare To Constant/1 -> Data Type Conversion/1
  Data Store Read8/1 -> CIRCUIT/Enable
  Data Store Read13/1 -> Bus Assignment1/1
  CIRCUIT/3(d_sens (m)) -> Bus Assignment1/4
  CIRCUIT/5(estado) -> Bus Assignment1/6
  CIRCUIT/2(theta_circ (rad)) -> Bus Assignment1/3
  Bus Assignment1/1 -> Data Store Write1/1
  Data Store Read3/1 -> Demux/1
  CIRCUIT/4(rampa) -> Bus Assignment1/5
  CIRCUIT/1(dist (mm)) -> Bus Assignment1/2
  Data Store Read15/1 -> CIRCUIT/3(theta (rad))
  Demux/2 -> CIRCUIT/2(yA)
  Demux/1 -> CIRCUIT/1(xA)
  Data Store Read16/1 -> CIRCUIT SIMULATION/1(MODEL_IN)
  CIRCUIT SIMULATION/1(MODEL) -> Data Store Write6/1
  ACCELERATION RATE/1(REAL MOTOR VOLT) -> Data Store Write7/1
  Data Store Read6/1 -> ACCELERATION RATE/1(CONTROL MOTOR VOLT)
  Data Store Read17/1 -> ACCELERATION RATE/2(MOTOR VOLT MAX)
  Bus Selector/1 -> Data Type Conversion1/1  "<COMP_FINISHED>"
  Data Type Conversion1/1 -> Stop Simulation/1
  Data Store Read11/1 -> Bus Selector/1, SENSOR MODEL/2(CONTROL_IN)
  ? -> ?
  MCS DELAY/1(CONTROL_OUT) -> Data Store Write3/1

== system TEST_LIDAR/COMPUTATIONAL LOAD/Accumulator 1 ==
  In : Inport
  Memory : Memory  InheritSampleTime=on
  Sum1 : Sum  Inputs=|++  AccumDataTypeStr=uint32  OutDataTypeStr=uint32
  Sum : Outport  VectorParamsAs1DForOutWhenUnconnected=off
  wires:
  In/1 -> Sum1/1
  Sum1/1 -> Memory/1
  Memory/1 -> Sum/1, Sum1/2

== system TEST_LIDAR/COMPUTATIONAL LOAD/Accumulator 2 ==
  In : Inport
  Memory : Memory  InheritSampleTime=on
  Sum1 : Sum  Inputs=|++  AccumDataTypeStr=uint32  OutDataTypeStr=uint32
  Sum : Outport  VectorParamsAs1DForOutWhenUnconnected=off
  wires:
  In/1 -> Sum1/1
  Sum1/1 -> Memory/1
  Memory/1 -> Sum/1, Sum1/2

== system TEST_LIDAR/COMPUTATIONAL LOAD/Accumulator 3 ==
  In : Inport
  Memory : Memory  InheritSampleTime=on
  Sum1 : Sum  Inputs=|++  AccumDataTypeStr=uint32  OutDataTypeStr=uint32
  Sum : Outport  VectorParamsAs1DForOutWhenUnconnected=off
  wires:
  In/1 -> Sum1/1
  Sum1/1 -> Memory/1
  Memory/1 -> Sum/1, Sum1/2

== system TEST_LIDAR/COMPUTATIONAL LOAD/Accumulator 4 ==
  In : Inport
  Memory : Memory  InheritSampleTime=on
  Sum1 : Sum  Inputs=|++  AccumDataTypeStr=uint32  OutDataTypeStr=uint32
  Sum : Outport  VectorParamsAs1DForOutWhenUnconnected=off
  wires:
  In/1 -> Sum1/1
  Sum1/1 -> Memory/1
  Memory/1 -> Sum/1, Sum1/2

== system TEST_LIDAR/CONTROL/ACCELERATION RATE ==
  CONTROL MOTOR VOLT : Inport
  MOTOR VOLT MAX : Inport  Port=2
  Demux : Demux  Outputs=2
  Gain : Gain  Gain=10/MD25.PWM_MAX/25e-3*SAMPLING_TIME
  Gain1 : Gain  Gain=0.5
  Gain2 : Gain  Gain=-1
  Gain3 : Gain  Gain=-1
  Gain4 : Gain  Gain=0.5
  Mux : Mux  Inputs=2
  Quantizer : Quantizer  QuantizationInterval=CONTROL_INI.PARAM.MOTOR_VOLT_MAX(1)/127
  Saturation Dynamic : simulink/Discontinuities/Saturation Dynamic  OutMin=[]  OutMax=[]  OutDataTypeStr=Inherit: Same as second input  OutDataType=fixdt(1, 16)  OutScaling=2^-10  DoSatur=off
  Saturation Dynamic1 : simulink/Discontinuities/Saturation Dynamic  OutMin=[]  OutMax=[]  OutDataTypeStr=Inherit: Same as second input  OutDataType=fixdt(1, 16)  OutScaling=2^-10  DoSatur=off
  Sum : Sum  Inputs=|+-
  Sum1 : Sum  Inputs=|++
  Sum2 : Sum  Inputs=|++
  Sum3 : Sum  Inputs=+-|
  Unit Delay1 : UnitDelay  SampleTime=-1  HasFrameUpgradeWarning=on
  REAL MOTOR VOLT : Outport
  REAL MOTOR VOLT_CD : Outport  Port=2
  wires:
  CONTROL MOTOR VOLT/1 -> Quantizer/1
  Gain3/1 -> Saturation Dynamic1/3
  Gain2/1 -> Saturation Dynamic/3
  Sum/1 -> Saturation Dynamic/2
  MOTOR VOLT MAX/1 -> Gain/1, Gain3/1, Saturation Dynamic1/1
  Sum1/1 -> Saturation Dynamic1/2
  Gain/1 -> Gain2/1, Saturation Dynamic/1
  Saturation Dynamic/1 -> Sum1/1
  Saturation Dynamic1/1 -> Unit Delay1/1, Demux/1, REAL MOTOR VOLT/1
  Demux/1 -> Sum3/1, Sum2/1
  Demux/2 -> Sum3/2, Sum2/2
  Sum2/1 -> Gain1/1
  Sum3/1 -> Gain4/1
  Gain1/1 -> Mux/1
  Gain4/1 -> Mux/2
  Mux/1 -> REAL MOTOR VOLT_CD/1
  Unit Delay1/1 -> Sum/2, Sum1/2
  Quantizer/1 -> Sum/1

== system TEST_LIDAR/CONTROL/ADAPTIVE CONTROL STR ==
  VEL_PARAM : Inport
  Enable : EnablePort
  Data Store Read : DataStoreRead  DataStoreName=CONTROL  SampleTime=SAMPLING_TIME  DataStoreElements=CONTROL.PARAM.FORWARD_VEL_PID.K#CONTROL.PARAM.FORWARD_VEL_PID.Ti#CONTROL.PARAM.FORWARD_VEL_PID.b  IndexOptions=Index vector (dialog)  Indices=1  OutputSizes=1
  Data Store Read2 : DataStoreRead  DataStoreName=CONTROL  SampleTime=SAMPLING_TIME  IndexOptions=Index vector (dialog)  Indices=1  OutputSizes=1
  Data Store Write : DataStoreWrite  DataStoreName=CONTROL  DataStoreElements=CONTROL.PARAM.FORWARD_VEL_PID.K#CONTROL.PARAM.FORWARD_VEL_PID.Ti#CONTROL.PARAM.FORWARD_VEL_PID.b  IndexOptions=Index vector (dialog)  Indices=1  OutputSizes=1
  Data Store Write1 : DataStoreWrite  DataStoreName=CONTROL  DataStoreElements=CONTROL.PARAM.FV_PI_STR_K#CONTROL.PARAM.FV_PI_STR_Ti#CONTROL.PARAM.FV_PI_STR_b#CONTROL.PARAM.ADPT_FLAG  IndexOptions=Index vector (dialog)  Indices=1  OutputSizes=1
  Data Type Conversion : DataTypeConversion  OutDataTypeStr=uint8  SaturateOnIntegerOverflow=off  RndMeth=Floor
  Delay : Delay  DelayLength=1  InitialConditionSource=Input port
      settings: InputPortMap=u0,p4
  Delay1 : Delay  DelayLength=1  InitialConditionSource=Input port
      settings: InputPortMap=u0,p4
  Delay2 : Delay  DelayLength=1  InitialConditionSource=Input port
      settings: InputPortMap=u0,p4
  Display{,1..6} (7 alike) : Display
  PI DESIGN : MATLAB Function  TreatAsAtomicUnit=on
  Scope : Scope  NumInputPorts=4
  Switch : Switch  Criteria=u2 > Threshold  SaturateOnIntegerOverflow=off  InputSameDT=off
  Switch1 : Switch  Criteria=u2 > Threshold  SaturateOnIntegerOverflow=off  InputSameDT=off
  Switch2 : Switch  Criteria=u2 > Threshold  SaturateOnIntegerOverflow=off  InputSameDT=off
  wires:
  VEL_PARAM/1 -> PI DESIGN/1(PARAM)
  PI DESIGN/1(K_out) -> Display/1, Scope/1, Switch/1, Data Store Write1/1
  PI DESIGN/3(b_out) -> Scope/3, Display2/1, Switch2/1, Data Store Write1/3
  PI DESIGN/2(Ti_out) -> Display1/1, Scope/2, Switch1/1, Data Store Write1/2
  Switch/1 -> Display6/1, Data Store Write/1
  Switch2/1 -> Data Store Write/3, Display4/1
  Switch1/1 -> Data Store Write/2, Display5/1
  Data Store Read/1 -> Delay2/2, Delay2/1
  Data Store Read/2 -> Delay1/1, Delay1/2
  Delay/1 -> Switch2/3
  Delay1/1 -> Switch1/3
  Delay2/1 -> Switch/3
  PI DESIGN/4(FLAG_ADPT_out) -> Display3/1, Scope/4, Switch/2, Switch1/2, Switch2/2, Data Type Conversion/1
  Data Store Read/3 -> Delay/1, Delay/2
  Data Store Read2/1 -> PI DESIGN/2(CONTROL)
  Data Type Conversion/1 -> Data Store Write1/4

== system TEST_LIDAR/CONTROL/LOCAL TARGETS ==
  Enable : EnablePort
  Compare To Constant1 : simulink/Logic and Bit Operations/Compare To Constant  relop===  const=4  OutDataTypeStr=boolean
  Compare To Constant10 : simulink/Logic and Bit Operations/Compare To Constant  relop===  const=10  OutDataTypeStr=boolean
  Compare To Constant11 : simulink/Logic and Bit Operations/Compare To Constant  relop===  const=9  OutDataTypeStr=boolean
  Compare To Constant12 : simulink/Logic and Bit Operations/Compare To Constant  relop===  const=6  OutDataTypeStr=boolean
  Compare To Constant2 : simulink/Logic and Bit Operations/Compare To Constant  relop===  const=5  OutDataTypeStr=boolean
  Compare To Constant3 : simulink/Logic and Bit Operations/Compare To Constant  relop===  const=7  OutDataTypeStr=boolean
  Compare To Constant4 : simulink/Logic and Bit Operations/Compare To Constant  relop===  const=5  OutDataTypeStr=boolean
  Compare To Constant5 : simulink/Logic and Bit Operations/Compare To Constant  relop===  const=3  OutDataTypeStr=boolean
  Compare To Constant6 : simulink/Logic and Bit Operations/Compare To Constant  relop===  const=4  OutDataTypeStr=boolean
  Compare To Constant7 : simulink/Logic and Bit Operations/Compare To Constant  relop===  const=7  OutDataTypeStr=boolean
  Compare To Constant8 : simulink/Logic and Bit Operations/Compare To Constant  relop===  const=8  OutDataTypeStr=boolean
  Compare To Constant9 : simulink/Logic and Bit Operations/Compare To Constant  relop===  const=8  OutDataTypeStr=boolean
  Data Store Read{1..5,8} (6 alike) : DataStoreRead  DataStoreName=CONTROL  SampleTime=SAMPLING_TIME  DataStoreElements=CONTROL.STATE.CURRENT_STATUS_SYS  IndexOptions=Index vector (dialog)  Indices=1  OutputSizes=1
  FORWARD VELOCITY TARGET : Subsystem
  Logical Operator : Logic  Operator=OR  Inputs=5  AllPortsSameDT=off  OutDataTypeStr=boolean
  Logical Operator1 : Logic  Operator=OR  AllPortsSameDT=off  OutDataTypeStr=boolean
  Logical Operator2 : Logic  Operator=OR  AllPortsSameDT=off  OutDataTypeStr=boolean
  NAVIGATION TARGETS : Subsystem  Priority=10
      settings: MinAlgLoopOccurrences=on
  OPL TARGETS : Subsystem
  WFL TARGETS : Subsystem
  YAW ANGLE TARGET : Subsystem
  YAW RATE TARGET : Subsystem
  wires:
  Compare To Constant5/1 -> OPL TARGETS/Enable
  Data Store Read8/1 -> Compare To Constant5/1
  Data Store Read2/1 -> Compare To Constant10/1, Compare To Constant8/1, Compare To Constant7/1, Compare To Constant6/1, Compare To Constant2/1
  Data Store Read3/1 -> Compare To Constant9/1, Compare To Constant3/1
  Data Store Read4/1 -> Compare To Constant4/1
  Compare To Constant4/1 -> YAW RATE TARGET/Enable
  Compare To Constant6/1 -> Logical Operator/1
  Compare To Constant2/1 -> Logical Operator/2
  Logical Operator/1 -> FORWARD VELOCITY TARGET/Enable
  Compare To Constant7/1 -> Logical Operator/3
  Compare To Constant8/1 -> Logical Operator/4
  Logical Operator1/1 -> WFL TARGETS/Enable
  Compare To Constant3/1 -> Logical Operator1/1
  Compare To Constant9/1 -> Logical Operator1/2
  Compare To Constant10/1 -> Logical Operator/5
  Compare To Constant1/1 -> YAW ANGLE TARGET/Enable
  Data Store Read1/1 -> Compare To Constant1/1
  Logical Operator2/1 -> NAVIGATION TARGETS/Enable
  Compare To Constant11/1 -> Logical Operator2/2
  Compare To Constant12/1 -> Logical Operator2/1
  Data Store Read5/1 -> Compare To Constant11/1, Compare To Constant12/1

== system TEST_LIDAR/CONTROL/MOTOR DELAY ==
  MOTOR_VOLT : Inport
  MOTOR_VOLT_CD : Inport  Port=2
  Compare To Constant4 : simulink/Logic and Bit Operations/Compare To Constant  relop===  const=1  OutDataTypeStr=boolean
  Data Store Read1 : DataStoreRead  DataStoreName=CONTROL  SampleTime=SAMPLING_TIME  DataStoreElements=CONTROL.PARAM.SAMPLING_TIME  IndexOptions=Index vector (dialog)  Indices=1  OutputSizes=1
  Data Store Read11 : DataStoreRead  DataStoreName=CONTROL  SampleTime=SAMPLING_TIME  DataStoreElements=CONTROL.STATE.MOTOR_DELAY_MODE  IndexOptions=Index vector (dialog)  Indices=1  OutputSizes=1
  Data Store Read2 : DataStoreRead  DataStoreName=CONTROL  SampleTime=SAMPLING_TIME  DataStoreElements=CONTROL.PARAM.MOTOR_DELAY_ERR  IndexOptions=Index vector (dialog)  Indices=1  OutputSizes=1
  Data Store Read6 : DataStoreRead  DataStoreName=CONTROL  SampleTime=SAMPLING_TIME  DataStoreElements=CONTROL.PARAM.MOTOR_DELAY  IndexOptions=Index vector (dialog)  Indices=1  OutputSizes=1
  Data Store Write1 : DataStoreWrite  DataStoreName=CONTROL  DataStoreElements=CONTROL.OUTPUT.MOTOR_VOLT_CD(:,:)  IndexOptions=Index vector (dialog)  Indices=1  OutputSizes=1
  Data Store Write4 : DataStoreWrite  DataStoreName=CONTROL  DataStoreElements=CONTROL.OUTPUT.MOTOR_VOLT(:,:)  IndexOptions=Index vector (dialog)  Indices=1  OutputSizes=1
  Data Type Conversion : DataTypeConversion  OutDataTypeStr=double  SaturateOnIntegerOverflow=off  RndMeth=Floor
  Delay : Delay  DelayLengthSource=Input port  DelayLengthUpperLimit=20  SampleTime=SAMPLING_TIME
      settings: InputPortMap=u0,p1
  Delay1 : Delay  DelayLengthSource=Input port  DelayLengthUpperLimit=20  SampleTime=SAMPLING_TIME
      settings: InputPortMap=u0,p1
  Product : Product  Inputs=*/*
  Rounding Function : Rounding
  Sum : Sum  Inputs=++|
  wires:
  Delay/1 -> Data Store Write4/1
  Rounding Function/1 -> Delay1/2, Delay/2
  Product/1 -> Rounding Function/1
  Data Store Read1/1 -> Product/2
  Data Store Read6/1 -> Sum/2
  Sum/1 -> Product/1
  Data Store Read2/1 -> Sum/1
  Delay1/1 -> Data Store Write1/1
  MOTOR_VOLT_CD/1 -> Delay1/1
  Data Store Read11/1 -> Compare To Constant4/1
  Compare To Constant4/1 -> Data Type Conversion/1
  Data Type Conversion/1 -> Product/3
  MOTOR_VOLT/1 -> Delay/1
